simulink model "sym4"  (R2022b)
settings: Solver=VariableStepAuto  StartTime=0.0  StopTime=100  RelTol=1e-3
values from neighbouring files (symbols this model uses):
  Hdc1 = minreal(Haux1/Haux2)    [Lab4.m]
  Hdc2 = minreal(Hdc1*tf([1 -ZPKHdc1.P{1,1}(4)], 1, Ts, 'Variable', 'z^-1'))    [Lab4.m]
  Hf = tf(Kp, [T1*T2 T1+T2 1], 'IoDelay', Tm)    [Lab4.m]
  k = 5    [Lab4.m]
  Ts = Tm/k    (= 0.5)    [Lab4.m]
settings Model: Creator=Pacuraru Fabian  LastModifiedBy=Pacuraru Fabian

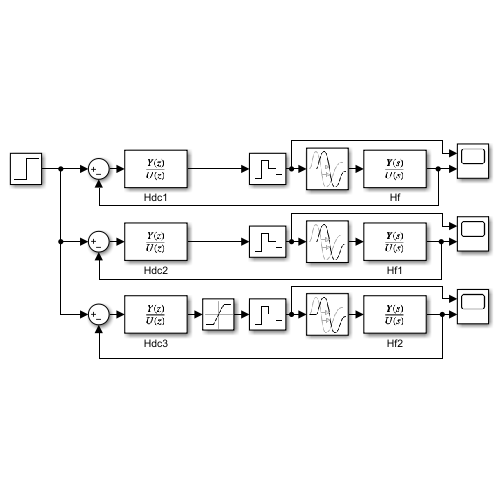
[thumbnail: Simulink's stored preview of the top-level diagram]
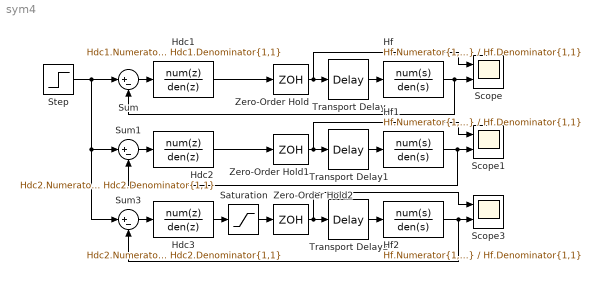
== system sym4 ==
  Hdc1 : DiscreteTransferFcn  Numerator=Hdc1.Numerator{1,1}  Denominator=Hdc1.Denominator{1,1}  SampleTime=Ts
  Hdc2 : DiscreteTransferFcn  Numerator=Hdc2.Numerator{1,1}  Denominator=Hdc2.Denominator{1,1}  SampleTime=Ts
  Hdc3 : DiscreteTransferFcn  Numerator=Hdc2.Numerator{1,1}  Denominator=Hdc2.Denominator{1,1}  SampleTime=Ts
  Hf : TransferFcn  Numerator=Hf.Numerator{1,1}  Denominator=Hf.Denominator{1,1}
  Hf1 : TransferFcn  Numerator=Hf.Numerator{1,1}  Denominator=Hf.Denominator{1,1}
  Hf2 : TransferFcn  Numerator=Hf.Numerator{1,1}  Denominator=Hf.Denominator{1,1}
  Saturation : Saturate  UpperLimit=1  LowerLimit=0
  Scope : Scope  NumInputPorts=2
  Scope1 : Scope  NumInputPorts=2
  Scope3 : Scope  NumInputPorts=2
  Step : Step  Time=0  SampleTime=0
  Sum : Sum  Inputs=|+-
  Sum1 : Sum  Inputs=|+-
  Sum3 : Sum  Inputs=|+-
  Transport Delay : TransportDelay  DelayTime=k
  Transport Delay1 : TransportDelay  DelayTime=k
  Transport Delay2 : TransportDelay  DelayTime=k
  Zero-Order Hold : ZeroOrderHold  SampleTime=Ts
  Zero-Order Hold1 : ZeroOrderHold  SampleTime=Ts
  Zero-Order Hold2 : ZeroOrderHold  SampleTime=Ts
  wires:
  Hf/1 -> Sum/2, Scope/2
  Sum/1 -> Hdc1/1
  Hf1/1 -> Sum1/2, Scope1/2
  Sum1/1 -> Hdc2/1
  Step/1 -> Sum3/1, Sum1/1, Sum/1
  Hf2/1 -> Sum3/2, Scope3/2
  Sum3/1 -> Hdc3/1
  Hdc1/1 -> Zero-Order Hold/1
  Hdc2/1 -> Zero-Order Hold1/1
  Zero-Order Hold/1 -> Transport Delay/1, Scope/1
  Transport Delay/1 -> Hf/1
  Zero-Order Hold1/1 -> Scope1/1, Transport Delay1/1
  Transport Delay1/1 -> Hf1/1
  Transport Delay2/1 -> Hf2/1
  Zero-Order Hold2/1 -> Scope3/1, Transport Delay2/1
  Hdc3/1 -> Saturation/1
  Saturation/1 -> Zero-Order Hold2/1
